simulink model "FunctionQ1"  (R2020b)
settings: Solver=VariableStepAuto  StartTime=0.0  StopTime=30  RelTol=1e-3
settings Model: Creator=Javad  LastModifiedBy=Javad

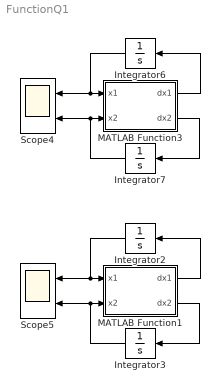
== system FunctionQ1 ==
  Integrator2 : Integrator  InitialCondition=3
  Integrator3 : Integrator  InitialCondition=5
  Integrator6 : Integrator  InitialCondition=3
  Integrator7 : Integrator  InitialCondition=5
  MATLAB Function1 : MATLAB Function  TreatAsAtomicUnit=on
  MATLAB Function3 : MATLAB Function  TreatAsAtomicUnit=on
  Scope4 : Scope  NumInputPorts=2
  Scope5 : Scope  NumInputPorts=2
  wires:
  Integrator2/1 -> Scope5/1, MATLAB Function1/1(x1)
  MATLAB Function1/2(dx2) -> Integrator3/1
  MATLAB Function1/1(dx1) -> Integrator2/1
  Integrator3/1 -> Scope5/2, MATLAB Function1/2(x2)
  Integrator6/1 -> Scope4/1, MATLAB Function3/1(x1)
  MATLAB Function3/2(dx2) -> Integrator7/1
  MATLAB Function3/1(dx1) -> Integrator6/1
  Integrator7/1 -> Scope4/2, MATLAB Function3/2(x2)

== matlab function FunctionQ1/MATLAB Function3 ==
  data: x1 input; dx1 output; x2 input; dx2 output
function [dx1,dx2] = fcn2(x1,x2)
c=100;
dx1=-tanh(c*x1)+2*tanh(c*x2);
dx2=-2*tanh(c*x1)-tanh(c*x2);

== matlab function FunctionQ1/MATLAB Function1 ==
  data: x1 input; dx1 output; x2 input; dx2 output
function [dx1,dx2] = fcn3(x1,x2)
c=1;
dx1=-sign(c*x1)+2*sign(c*x2);
dx2=-2*sign(c*x1)-sign(c*x2);
